simulink model "simple"  (Simulink 6.4)
settings: Solver=ode23  StartTime=0.0  StopTime=20.0  RelTol=1e-3
settings Model: LastModifiedBy=crr501  ExtModeTrigMode=oneshot  ExtModeArmWhenConnect=off
settings DataIOCC: LimitDataPoints=off
settings OptimizationCC: BlockReduction=off  BooleanDataType=off
settings DebuggingCC: SolverPrmCheckMsg=none  StrictBusMsg=None
settings HardwareCC: TargetUnknown=on
settings STFCustomTargetCC: TargetFcnLib=ansi_tfl_tmw.mat  GenFloatMathFcnCalls=ANSI_C  ModelReferenceCompliant=off  IncludeERTFirstTime=on  SystemTargetFile=grt.tlc

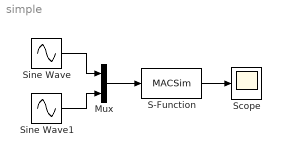
== system simple ==
  Mux : Mux  Inputs=2
  S-Function : S-Function  FunctionName=MACSim
  Scope : Scope
  Sine Wave : Sin  SampleTime=0
  Sine Wave1 : Sin  Frequency=4  SampleTime=0
  wires:
  Mux/1 -> S-Function/1
  Sine Wave1/1 -> Mux/2
  Sine Wave/1 -> Mux/1
  S-Function/1 -> Scope/1
